simulink model "ManuscriptID_9579_1"  (R2022b)
settings: Solver=ode45  StartTime=0.0  StopTime=2  RelTol=1e-3  EnableMultiTasking=on
libraries: spsVoltageMeasurementLib x10, spsIGBTDiodeLib x9, spsSeriesRLCBranchLib x5, spsCurrentMeasurementLib x2, spsDCVoltageSourceLib x2, sps_lib x1
settings Model: Creator=dhanu  LastModifiedBy=dell
settings SolverCC: AlgebraicLoopSolver=TrustRegion
settings DataIOCC: LimitDataPoints=on  SaveFormat=Array  ReturnWorkspaceOutputs=off
settings OptimizationCC: LifeSpan=inf
settings DebuggingCC: UnderspecifiedInitializationDetection=Classic  MergeDetectMultiDrivingBlocksExec=none  SolverPrmCheckMsg=warning  UnconnectedInputMsg=warning  UnconnectedOutputMsg=warning  UnconnectedLineMsg=warning  StateNameClashWarn=warning  SFUnexpectedBacktrackingDiag=warning  SFNoUnconditionalDefaultTransitionDiag=warning  SFExecutionAtInitializationDiag=none  SFMachineParentedDataDiag=warning  ArithmeticOperatorsInVariantConditions=warning
settings HardwareCC: ProdBitPerPointer=32  ProdBitPerSizeT=32  ProdBitPerPtrDiffT=32  ProdLargestAtomicFloat=None  ProdIntDivRoundTo=Undefined  ProdEndianess=Unspecified  ProdWordSize=32  ProdHWDeviceType=32-bit Generic
settings ModelReferenceCC: PropagateSignalLabelsOutOfModel=off
settings SFSimCC: SimUseLocalCustomCode=off  CustomCodeUndefinedFunction=UseInterfaceOnly
settings RTWCC: RTWUseLocalCustomCode=off
settings CodeAppCC: StateflowObjectComments=on
settings GRTTargetCC: TargetLangStandard=C89/C90 (ANSI)
settings ConfigComp: CovMetricSettings=dw  CovSaveCumulativeToWorkspaceVar=on  CovSaveSingleToWorkspaceVar=on  CovExternalEMLEnable=off
settings SimscapeCC: SimscapeNormalizeSystem=off

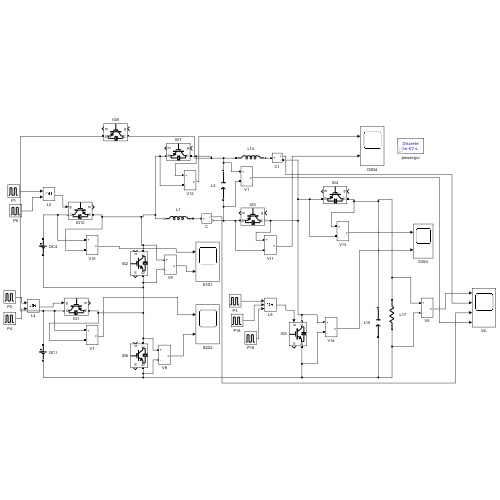
[thumbnail: Simulink's stored preview of the top-level diagram]
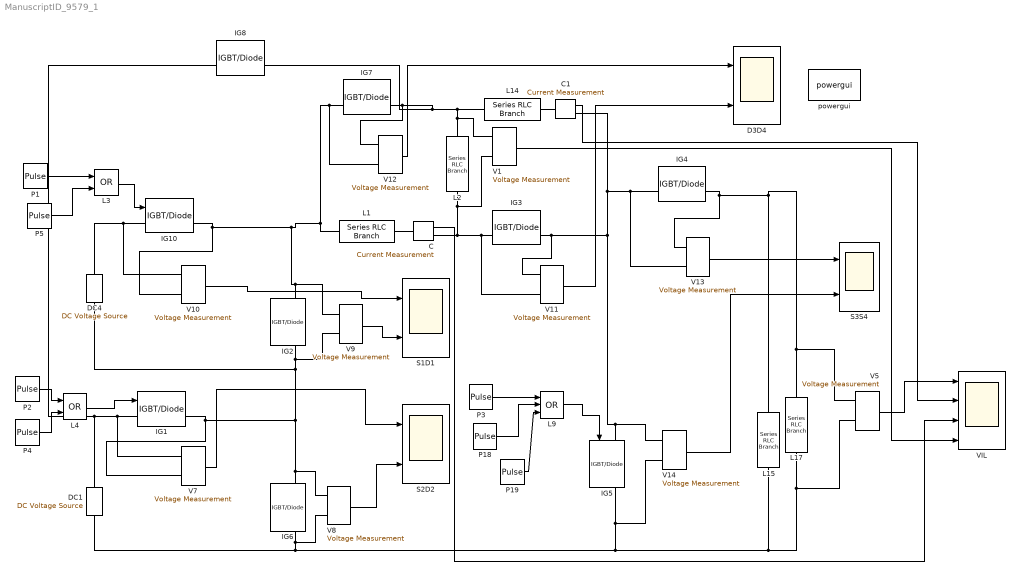
== system ManuscriptID_9579_1 ==
  C : spsCurrentMeasurementLib/Current Measurement  PhasorSimulation=off  OutputType=Complex  PSBequivalent=0
  C1 : spsCurrentMeasurementLib/Current Measurement  PhasorSimulation=off  OutputType=Complex  PSBequivalent=0
  D3D4 : Scope  NumInputPorts=2
  DC1 : spsDCVoltageSourceLib/DC Voltage Source  Amplitude=10  Measurements=None
  DC4 : spsDCVoltageSourceLib/DC Voltage Source  Amplitude=20  Measurements=None
  IG{1..8,10} (9 alike) : spsIGBTDiodeLib/IGBT//Diode  Ron=1e-3  Rs=1e5  Cs=inf  Measurements=on
  L1 : spsSeriesRLCBranchLib/Series RLC Branch  LConnTagsString=__new0  RConnTagsString=__new0  BranchType=L  Resistance=1  Inductance=4e-3  SetiL0=off  InitialCurrent=0  Capacitance=1e-6  Setx0=off  InitialVoltage=0  Measurements=None
  L14 : spsSeriesRLCBranchLib/Series RLC Branch  LConnTagsString=__new0  RConnTagsString=__new0  BranchType=L  Resistance=1  Inductance=4e-3  SetiL0=off  InitialCurrent=0  Capacitance=1e-6  Setx0=off  InitialVoltage=0  Measurements=None
  L15 : spsSeriesRLCBranchLib/Series RLC Branch  LConnTagsString=__new0  RConnTagsString=__new0  BranchType=C  Resistance=1  Inductance=1e-3  SetiL0=off  InitialCurrent=0  Capacitance=470e-6  Setx0=off  InitialVoltage=0  Measurements=None
  L17 : spsSeriesRLCBranchLib/Series RLC Branch  LConnTagsString=__new0  RConnTagsString=__new0  BranchType=R  Resistance=80  Inductance=1e-3  SetiL0=off  InitialCurrent=0  Capacitance=1000e-6  Setx0=off  InitialVoltage=0  Measurements=None
  L2 : spsSeriesRLCBranchLib/Series RLC Branch  LConnTagsString=__new0  RConnTagsString=__new0  BranchType=C  Resistance=1  Inductance=1e-3  SetiL0=off  InitialCurrent=0  Capacitance=360e-6  Setx0=off  InitialVoltage=0  Measurements=None
  L3 : Logic  Operator=OR  AllPortsSameDT=off  OutDataTypeStr=boolean
  L4 : Logic  Operator=OR  AllPortsSameDT=off  OutDataTypeStr=boolean
  L9 : Logic  Operator=OR  Inputs=3  AllPortsSameDT=off  OutDataTypeStr=boolean
  P1 : DiscretePulseGenerator  PulseType=Time based  Amplitude=15  Period=1/10000  PulseWidth=30
  P18 : DiscretePulseGenerator  PulseType=Time based  Amplitude=15  Period=1/10000  PulseWidth=30  PhaseDelay=0.000031
  P19 : DiscretePulseGenerator  PulseType=Time based  Amplitude=15  Period=1/10000  PulseWidth=10  PhaseDelay=0.000061
  P2 : DiscretePulseGenerator  PulseType=Time based  Amplitude=15  Period=1/10000  PulseWidth=10  PhaseDelay=0.000061
  P3 : DiscretePulseGenerator  PulseType=Time based  Amplitude=15  Period=1/10000  PulseWidth=30
  P4 : DiscretePulseGenerator  PulseType=Time based  Amplitude=15  Period=1/10000  PulseWidth=30  PhaseDelay=0.000031
  P5 : DiscretePulseGenerator  PulseType=Time based  Amplitude=15  Period=1/10000  PulseWidth=25  PhaseDelay=0.000031
  S1D1 : Scope  NumInputPorts=2
  S2D2 : Scope  NumInputPorts=2
  S3S4 : Scope  NumInputPorts=2
  V{1,5,7..14} (10 alike) : spsVoltageMeasurementLib/Voltage Measurement  PhasorSimulation=off  OutputType=Complex  PSBequivalent=0
  VIL : Scope  NumInputPorts=4
  powergui : sps_lib/powergui  Priority=1  SimulationMode=Discrete  SampleTime=50e-8  frequency=60  Iterations=50  frequencyindice=0  Pbase=100e6  ErrMax=1e-4  UnitsV=kV  UnitsW=MW  buscounter=0  FunctionMessages=off  echomessages=off  EnableUseOfTLC=off  CurrentSourceSwitches=off  DisableSnubberDevices=off  DisableRonSwitches=off  DisableVfSwitches=off  DisplayEquations=off  AutomaticDiscreteSolvers=off  SolverType=Tustin  Interpol=off  ExternalGateDelay=off  methode=off  Ts=0  x0status=blocks  SPID=off  SwTol=0  HookPort=off  NonlinearTolerance=1e-4  nMaxIteration=100  ContinueOnMaxIteration=off  RestoreLinks=warning  ResistiveCurrentMeasurement=off  Frange=[0:2:500]  Ylog=off  Xlog=on  ShowGrid=off  save=off  variable=ZData  structure=0  ZoomFFT=off  StartTime=0.0  cycles=1  DisplayStyle=1  fundamental=60  FreqAxis=off  MaxFrequency=1000  frequencyindicesteady=1  RmsSteady=1  display=off
  wires:
  P1/1 -> L3/1
  L3/1 -> IG10/1
  P2/1 -> L4/1
  L4/1 -> IG1/1
  P4/1 -> L4/2
  P5/1 -> L3/2
  V7/1 -> S2D2/1
  V8/1 -> S2D2/2
  V10/1 -> S1D1/1
  V9/1 -> S1D1/2
  V12/1 -> D3D4/1
  V11/1 -> D3D4/2
  V13/1 -> S3S4/1
  V14/1 -> S3S4/2
  V5/1 -> VIL/1
  C/1 -> VIL/3
  V1/1 -> VIL/4
  C1/1 -> VIL/2
  P18/1 -> L9/2
  L9/1 -> IG5/1
  P3/1 -> L9/1
  P19/1 -> L9/3
  connections:
  V13/LConn1 -- IG4/LConn1 -- V5/LConn1 -- L17/RConn1 -- L15/LConn1
  V8/LConn1 -- IG1/RConn1 -- V7/LConn2 -- DC4/LConn1 -- V9/LConn2 -- IG2/RConn1 -- IG6/LConn1
  IG1/LConn1 -- IG8/RConn1 -- DC1/RConn1 -- V7/LConn1
  L17/LConn1 -- V14/LConn2 -- IG5/RConn1 -- V8/LConn2 -- IG6/RConn1 -- DC1/LConn1 -- L15/RConn1 -- V5/LConn2
  V11/LConn1 -- V14/LConn1 -- IG5/LConn1 -- V13/LConn2 -- IG4/RConn1 -- C1/RConn1 -- IG3/LConn1
  DC4/RConn1 -- V10/LConn1 -- IG10/LConn1
  V12/LConn1 -- L14/RConn1 -- L2/LConn1 -- V1/LConn1 -- IG8/LConn1 -- IG7/LConn1
  L2/RConn1 -- C/RConn1 -- V11/LConn2 -- IG3/RConn1 -- V1/LConn2
  C/LConn1 -- L1/LConn1
  C1/LConn1 -- L14/LConn1
  IG2/LConn1 -- V9/LConn1 -- IG10/RConn1 -- V10/LConn2 -- IG7/RConn1 -- V12/LConn2 -- L1/RConn1
